simulink model "TP4_control_linealizante_perturbanciones"  (R2024b)
settings: Solver=VariableStepAuto  StartTime=0.0  StopTime=10.0  FixedStep=0.  RelTol=1e-3
undefined symbols (not defined in the file): e0, states0, v0
settings Model: Creator=tomii  LastModifiedBy=tomii

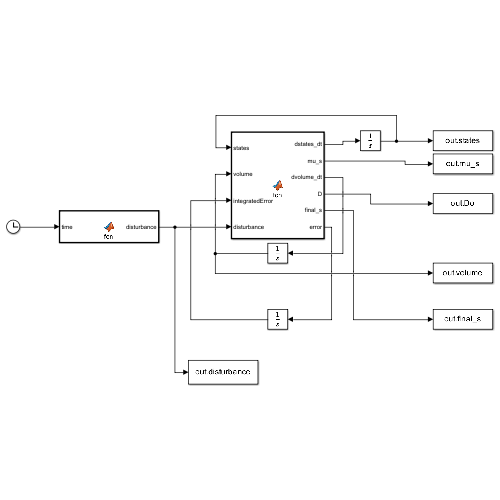
[thumbnail: Simulink's stored preview of the top-level diagram]
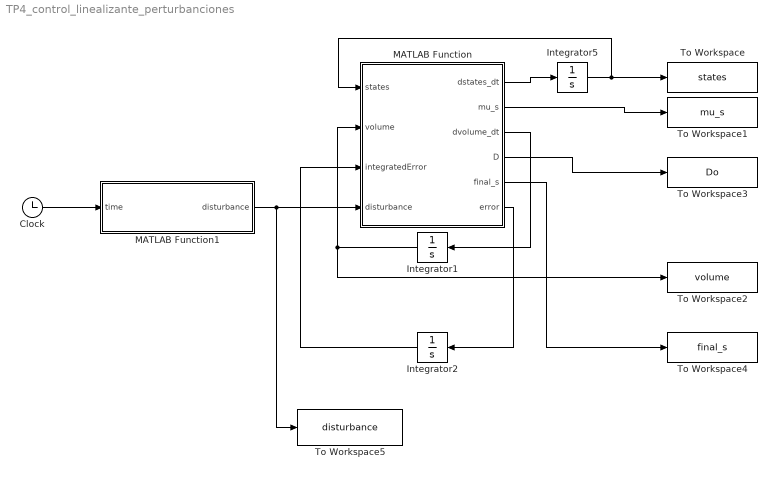
== system TP4_control_linealizante_perturbanciones ==
  Clock : Clock
  Integrator1 : Integrator  InitialCondition=v0
  Integrator2 : Integrator  InitialCondition=e0
  Integrator5 : Integrator  InitialCondition=states0
  MATLAB Function : MATLAB Function  TreatAsAtomicUnit=on
  MATLAB Function1 : MATLAB Function  TreatAsAtomicUnit=on
  To Workspace : ToWorkspace  VariableName=states  SaveFormat=Timeseries  SampleTime=-1
  To Workspace1 : ToWorkspace  VariableName=mu_s  SaveFormat=Timeseries  SampleTime=-1
  To Workspace2 : ToWorkspace  VariableName=volume  SaveFormat=Timeseries  SampleTime=-1
  To Workspace3 : ToWorkspace  VariableName=Do  SaveFormat=Timeseries  SampleTime=-1
  To Workspace4 : ToWorkspace  VariableName=final_s  SaveFormat=Timeseries  SampleTime=-1
  To Workspace5 : ToWorkspace  VariableName=disturbance  SaveFormat=Timeseries  SampleTime=-1
  wires:
  MATLAB Function/1(dstates_dt) -> Integrator5/1
  Integrator5/1 -> MATLAB Function/1(states), To Workspace/1
  MATLAB Function/2(mu_s) -> To Workspace1/1
  MATLAB Function/3(dvolume_dt) -> Integrator1/1
  Integrator1/1 -> MATLAB Function/2(volume), To Workspace2/1
  MATLAB Function/4(D) -> To Workspace3/1
  MATLAB Function/5(final_s) -> To Workspace4/1
  MATLAB Function/6(error) -> Integrator2/1
  Integrator2/1 -> MATLAB Function/3(integratedError)
  MATLAB Function1/1(disturbance) -> To Workspace5/1, MATLAB Function/4(disturbance)
  Clock/1 -> MATLAB Function1/1(time)

== matlab function TP4_control_linealizante_perturbanciones/MATLAB Function1 ==
  data: time input; disturbance output; disturbanceParameters parameter
function disturbance = fcn(time, disturbanceParameters)

    dStart = disturbanceParameters.start;
    dEnd = disturbanceParameters.end;
    percentage = disturbanceParameters.percentage;

    if (time > dEnd)
        disturbance = 0;
    elseif (time > dStart)
        disturbance = percentage;
    else
        disturbance = 0;
    end

end

== matlab function TP4_control_linealizante_perturbanciones/MATLAB Function ==
  data: dstates_dt output; mu_s output; states input; volume input; integratedError input; disturbance input; modelParameters parameter; dvolume_dt output; D output; final_s output; error output
function [dstates_dt, mu_s, dvolume_dt, D, final_s, error] = fcn(states, volume, integratedError, disturbance, modelParameters)   
    
    K=modelParameters.K;
    xi_in=modelParameters.xi_in;
    ks1=modelParameters.ks1;
    kp=modelParameters.kp;
    ki=modelParameters.ki;

    s_r=modelParameters.s_r;
    s_in=modelParameters.s_in;

    Ks=modelParameters.mu_model.Ks;
    Kis=modelParameters.mu_model.Kis;
    Kn=modelParameters.mu_model.Kn;
    mu_max=modelParameters.mu_model.mu_max;

    x=states(1);
    s=states(2);

    mu_s=mu_max*(s/(Ks+s+s*s/Kis))*(1/Kn);
    rx=x*mu_s;

    error=s_r-s;
    D=((1+kp*error+ki*integratedError)*(x*ks1)/(s_in-s_r))*(disturbance+1);
    final_s=s_in-x*ks1;

    dstates_dt = K * rx + D*(xi_in-states);
    dvolume_dt = 0;

end
